simulink model "uz_FOC"  (R2021a)
settings: Solver=FixedStepDiscrete  StartTime=0.0  StopTime=50.0  FixedStep=0.00001  RelTol=1e-3  EnableMultiTasking=on
values from neighbouring files (symbols this model uses):
  d_d_TMS = 0.005    [uz_FOC_init.m]
  d_f_c = 100000    [uz_FOC_init.m]
  d_i_max = 10    [uz_FOC_init.m]
  d_i_min = -d_i_max    (= -10)    [uz_FOC_init.m]
  d_J_Coupling_M_E = 2e-6    (= 2e-06)    [uz_FOC_init.m]
  d_J_Coupling_M_Ms = 2e-20    [uz_FOC_init.m]
  d_J_Ms_L = d_J_Ms_M    (= 1.26363648e-05)    [uz_FOC_init.m]
  d_J_Ms_M = 0.5*0.5*((0.5*d_d_Ms)^4)*3.14*d_l_Ms*d_rho_Ms    (= 1.26363648e-05)    [uz_FOC_init.m]
  d_Ki_id = d_Kp_id/d_Tn_id    (= 2000)    [uz_FOC_init.m]
  d_Ki_iq = d_Kp_iq/d_Tn_iq    (= 2000)    [uz_FOC_init.m]
  d_Ki_n = d_Kp_n/d_Tn_n    (= 0.0864)    [uz_FOC_init.m]
  d_Kp_id = d_L_d / (4*1/d_f_c)    (= 6.75)    [uz_FOC_init.m]
  d_Kp_iq = d_L_q / (4*1/d_f_c)    (= 6.75)    [uz_FOC_init.m]
  d_Kp_n = 0.00864    [uz_FOC_init.m]
  d_L_d = d_L_ph_ph/2    (= 0.00027)    [uz_FOC_init.m]
  d_L_q = d_L_ph_ph/2    (= 0.00027)    [uz_FOC_init.m]
  d_p = 4    [uz_FOC_init.m]
  d_psi_pm = 0.0082    [uz_FOC_init.m]
  d_R_ph = d_R_ph_ph/2    (= 0.08)    [uz_FOC_init.m]
  d_y_max = 10    [uz_FOC_init.m]
  d_y_min = -d_y_max    (= -10)    [uz_FOC_init.m]
undefined symbols (not defined in the file or in its folder): i_d, i_q, para, u_d, u_q
libraries: fl_lib x44, nesl_utility x27, ee_lib x21, simulink x8, spsabctodq0Lib x2, spsdq0toabcLib x1, spsTriangleGeneratorLib x1
(part 2 of 3)

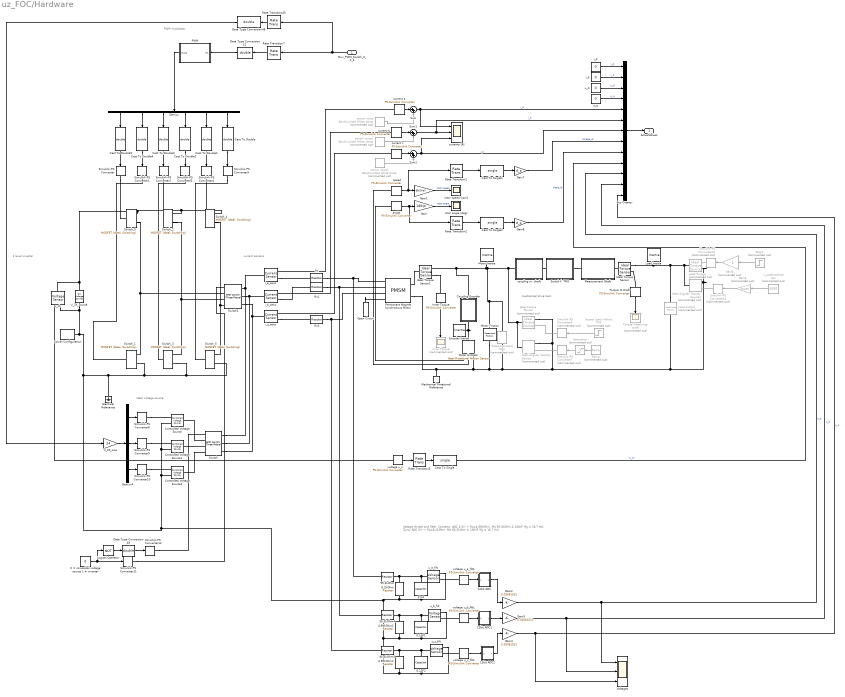
== system uz_FOC/Hardware ==
  note: PWM modulator
  note: 2 level inverter
  note: current sensors
  note: ideal voltage source
  note: Voltage divider and filter:
      | Concerto: ADC 3,3V -> RL=4,99kOhm. Mit 95,3kOhm & 100nF (fg = 16,7 Hz).
      | Zynq: ADC 5V -> RL=8,2kOhm. Mit 95,3kOhm & 100nF (fg = 16,7 Hz).
  note: mechanical drive train
  Mux_PWM_Switch_0_2_4 : Inport
  0 = sinusoidal voltage source 1 = inverter : Constant  Value=0
  0.1µF1 : ee_lib/Passive/Capacitor  cap_option=0  c=47 nF  Cvec=[ 1e-5 1e-6 ] F  Vvec=[ 0 10 ] V  CV_table_symmetry=1  f_vec=[1, 10] kHz  DFext_vec=[.8, 1.2]  C_tol=0.1  enable_C_tol=0  tol_distribution=1  nSigma=4  r=1e-18 Ohm  g=0 1/Ohm  averaging_period=0 s  enable_operating_limits=0  operating_limit_action=2  max_working_voltage_range=[ -25 25 ] V  power_rating=1 W  enable_faults=0  fault_action=1  Cscale_faulted=100  R_faulted=0.001 Ohm  G_faulted=0 1/Ohm  tau_fault=0.001 s  enable_temporal_fault=0  t_fault=1 s  enable_behavioral_fault=0  max_permissible_voltage_range=[ -100 100 ] V  t_fail_on_voltage=1 s  i_specify=off  i_priority=None  i=0 A  i_nominal_specify=off  i_nominal_unit=A  i_nominal_value=1  v_specify=off  v_priority=None  v=0 V  v_nominal_specify=off  v_nominal_unit=V  v_nominal_value=1  vc_specify=on  vc_priority=High  vc=0 V  vc_nominal_specify=off  vc_nominal_unit=V  vc_nominal_value=1
  0.1µF2 : ee_lib/Passive/Capacitor  cap_option=0  c=47 nF  Cvec=[ 1e-5 1e-6 ] F  Vvec=[ 0 10 ] V  CV_table_symmetry=1  f_vec=[1, 10] kHz  DFext_vec=[.8, 1.2]  C_tol=0.1  enable_C_tol=0  tol_distribution=1  nSigma=4  r=1e-18 Ohm  g=0 1/Ohm  averaging_period=0 s  enable_operating_limits=0  operating_limit_action=2  max_working_voltage_range=[ -25 25 ] V  power_rating=1 W  enable_faults=0  fault_action=1  Cscale_faulted=100  R_faulted=0.001 Ohm  G_faulted=0 1/Ohm  tau_fault=0.001 s  enable_temporal_fault=0  t_fault=1 s  enable_behavioral_fault=0  max_permissible_voltage_range=[ -100 100 ] V  t_fail_on_voltage=1 s  i_specify=off  i_priority=None  i=0 A  i_nominal_specify=off  i_nominal_unit=A  i_nominal_value=1  v_specify=off  v_priority=None  v=0 V  v_nominal_specify=off  v_nominal_unit=V  v_nominal_value=1  vc_specify=on  vc_priority=High  vc=0 V  vc_nominal_specify=off  vc_nominal_unit=V  vc_nominal_value=1
  12bit ADC : MATLAB Function  TreatAsAtomicUnit=on
  12bit ADC1 : MATLAB Function  TreatAsAtomicUnit=on
  12bit ADC2 : MATLAB Function  TreatAsAtomicUnit=on
  4,99kOhm1 : ee_lib/Passive/Resistor  R=8200 Ohm  R_tol=0.1  enable_R_tol=0  tol_distribution=1  nSigma=4  enable_operating_limits=0  operating_limit_action=2  max_working_voltage=100 V  power_rating=1 W  enable_faults=0  fault_action=1  R_faulted=Inf Ohm  enable_temporal_fault=0  t_fault=1 s  enable_behavioral_fault=0  max_permissible_current=1 A  t_fail_on_current=1 s  noise_mode=0  sample_time=0.001 s  repeatability=1  auto_seed=3032444857  user_seed=0  Tdevice=25 degC  alpha=3.93e-3 1/K  Tmeas=25 degC  thermal_mass=100 J/K  power_derating_T1=70 degC  power_derating_T2=155 degC  operating_temperature_range_vec=[-50, 150] degC  temperature_specify=off  temperature_priority=High  temperature=298.15 K  temperature_nominal_specify=off  temperature_nominal_unit=K  temperature_nominal_value=1
  4,99kOhm2 : ee_lib/Passive/Resistor  R=8200 Ohm  R_tol=0.1  enable_R_tol=0  tol_distribution=1  nSigma=4  enable_operating_limits=0  operating_limit_action=2  max_working_voltage=100 V  power_rating=1 W  enable_faults=0  fault_action=1  R_faulted=Inf Ohm  enable_temporal_fault=0  t_fault=1 s  enable_behavioral_fault=0  max_permissible_current=1 A  t_fail_on_current=1 s  noise_mode=0  sample_time=0.001 s  repeatability=1  auto_seed=136721035  user_seed=0  Tdevice=25 degC  alpha=3.93e-3 1/K  Tmeas=25 degC  thermal_mass=100 J/K  power_derating_T1=70 degC  power_derating_T2=155 degC  operating_temperature_range_vec=[-50, 150] degC  temperature_specify=off  temperature_priority=High  temperature=298.15 K  temperature_nominal_specify=off  temperature_nominal_unit=K  temperature_nominal_value=1
  47nF : ee_lib/Passive/Capacitor  cap_option=0  c=47 nF  Cvec=[ 1e-5 1e-6 ] F  Vvec=[ 0 10 ] V  CV_table_symmetry=1  f_vec=[1, 10] kHz  DFext_vec=[.8, 1.2]  C_tol=0.1  enable_C_tol=0  tol_distribution=1  nSigma=4  r=1e-20 Ohm  g=0 1/Ohm  averaging_period=0 s  enable_operating_limits=0  operating_limit_action=2  max_working_voltage_range=[ -25 25 ] V  power_rating=1 W  enable_faults=0  fault_action=1  Cscale_faulted=100  R_faulted=0.001 Ohm  G_faulted=0 1/Ohm  tau_fault=0.001 s  enable_temporal_fault=0  t_fault=1 s  enable_behavioral_fault=0  max_permissible_voltage_range=[ -100 100 ] V  t_fail_on_voltage=1 s  i_specify=off  i_priority=None  i=0 A  i_nominal_specify=off  i_nominal_unit=A  i_nominal_value=1  v_specify=off  v_priority=None  v=0 V  v_nominal_specify=off  v_nominal_unit=V  v_nominal_value=1  vc_specify=on  vc_priority=High  vc=0 V  vc_nominal_specify=off  vc_nominal_unit=V  vc_nominal_value=1
  8,2kOhm : ee_lib/Passive/Resistor  R=8200 Ohm  R_tol=0.1  enable_R_tol=0  tol_distribution=1  nSigma=4  enable_operating_limits=0  operating_limit_action=2  max_working_voltage=100 V  power_rating=1 W  enable_faults=0  fault_action=1  R_faulted=Inf Ohm  enable_temporal_fault=0  t_fault=1 s  enable_behavioral_fault=0  max_permissible_current=1 A  t_fail_on_current=1 s  noise_mode=0  sample_time=0.001 s  repeatability=1  auto_seed=1189375164  user_seed=0  Tdevice=25 degC  alpha=3.93e-3 1/K  Tmeas=25 degC  thermal_mass=100 J/K  power_derating_T1=70 degC  power_derating_T2=155 degC  operating_temperature_range_vec=[-50, 150] degC  temperature_specify=off  temperature_priority=High  temperature=298.15 K  temperature_nominal_specify=off  temperature_nominal_unit=K  temperature_nominal_value=1
  95,3kOhm : ee_lib/Passive/Resistor  R=95300 Ohm  R_tol=0.1  enable_R_tol=0  tol_distribution=1  nSigma=4  enable_operating_limits=0  operating_limit_action=2  max_working_voltage=100 V  power_rating=1 W  enable_faults=0  fault_action=1  R_faulted=Inf Ohm  enable_temporal_fault=0  t_fault=1 s  enable_behavioral_fault=0  max_permissible_current=1 A  t_fail_on_current=1 s  noise_mode=0  sample_time=0.001 s  repeatability=1  auto_seed=198304613  user_seed=0  Tdevice=25 degC  alpha=3.93e-3 1/K  Tmeas=25 degC  thermal_mass=100 J/K  power_derating_T1=70 degC  power_derating_T2=155 degC  operating_temperature_range_vec=[-50, 150] degC  temperature_specify=off  temperature_priority=High  temperature=298.15 K  temperature_nominal_specify=off  temperature_nominal_unit=K  temperature_nominal_value=1
  95,3kOhm4 : ee_lib/Passive/Resistor  R=95300 Ohm  R_tol=0.1  enable_R_tol=0  tol_distribution=1  nSigma=4  enable_operating_limits=0  operating_limit_action=2  max_working_voltage=100 V  power_rating=1 W  enable_faults=0  fault_action=1  R_faulted=Inf Ohm  enable_temporal_fault=0  t_fault=1 s  enable_behavioral_fault=0  max_permissible_current=1 A  t_fail_on_current=1 s  noise_mode=0  sample_time=0.001 s  repeatability=1  auto_seed=417177824  user_seed=0  Tdevice=25 degC  alpha=3.93e-3 1/K  Tmeas=25 degC  thermal_mass=100 J/K  power_derating_T1=70 degC  power_derating_T2=155 degC  operating_temperature_range_vec=[-50, 150] degC  temperature_specify=off  temperature_priority=High  temperature=298.15 K  temperature_nominal_specify=off  temperature_nominal_unit=K  temperature_nominal_value=1
  95,3kOhm5 : ee_lib/Passive/Resistor  R=95300 Ohm  R_tol=0.1  enable_R_tol=0  tol_distribution=1  nSigma=4  enable_operating_limits=0  operating_limit_action=2  max_working_voltage=100 V  power_rating=1 W  enable_faults=0  fault_action=1  R_faulted=Inf Ohm  enable_temporal_fault=0  t_fault=1 s  enable_behavioral_fault=0  max_permissible_current=1 A  t_fail_on_current=1 s  noise_mode=0  sample_time=0.001 s  repeatability=1  auto_seed=3536724442  user_seed=0  Tdevice=25 degC  alpha=3.93e-3 1/K  Tmeas=25 degC  thermal_mass=100 J/K  power_derating_T1=70 degC  power_derating_T2=155 degC  operating_temperature_range_vec=[-50, 150] degC  temperature_specify=off  temperature_priority=High  temperature=298.15 K  temperature_nominal_specify=off  temperature_nominal_unit=K  temperature_nominal_value=1
  Bus Creator : BusCreator  Inputs=13  OutDataTypeStr=Bus: ActualValues
  Cast To Double{,1..5} (6 alike) : DataTypeConversion  OutDataTypeStr=double
  Cast To Single : DataTypeConversion  OutDataTypeStr=single
  Cast To Single1 : DataTypeConversion  OutDataTypeStr=single
  Cast To Single2 : DataTypeConversion  OutDataTypeStr=single
  Controlled Voltage Source : fl_lib/Electrical/Electrical Sources/Controlled Voltage Source
  Controlled Voltage Source1 : fl_lib/Electrical/Electrical Sources/Controlled Voltage Source
  Controlled Voltage Source2 : fl_lib/Electrical/Electrical Sources/Controlled Voltage Source
  Coupling Encoder : Subsystem  Variant=on  VariantControlMode=label  LabelModeActiveChoice=TMS1
  Data Type Conversion12 : DataTypeConversion  OutDataTypeStr=double
  Data Type Conversion48 : DataTypeConversion  OutDataTypeStr=double
  Data Type Conversion49 : DataTypeConversion  OutDataTypeStr=double
  Demux : Demux  Outputs=6
  Demux4 : Demux  Outputs=3
  Electrical Reference : fl_lib/Electrical/Electrical Elements/Electrical Reference
  Encoder Inertia : fl_lib/Mechanical/Rotational Elements/Inertia  inertia=d_J_Encoder kg*m^2  num_ports=foundation.enum.numPorts2.one  w_specify=off  w_priority=High  w=0 rad/s  w_nominal_specify=off  w_nominal_unit=rad/s  w_nominal_value=1  t_specify=off  t_priority=None  t=0 N*m  t_nominal_specify=off  t_nominal_unit=N*m  t_nominal_value=1
  Gain : Gain  Gain=180/pi
  Gain1 : Gain  Gain=60/(2*pi)
  Gain2 : Gain  Gain=0.03081531  OutDataTypeStr=single
  Gain3 : Gain  Gain=0.03081531  OutDataTypeStr=single
  Gain4 : Gain  Gain=0.03081531  OutDataTypeStr=single
  Gain5 : Gain  Commented=on  Gain=-1
  Gain6 : Gain  Commented=on  Gain=2*pi/60
  Gain7 : Gain  Gain=d_p
  Gain8 : Gain  Gain=d_p
  Ideal Angular Velocity Source : fl_lib/Mechanical/Mechanical Sources/Ideal Angular Velocity Source  Commented=on
  Ideal Angular Velocity Source1 : fl_lib/Mechanical/Mechanical Sources/Ideal Angular Velocity Source  Commented=on
  Ideal Torque Sensor : fl_lib/Mechanical/Mechanical Sensors/Ideal Torque Sensor
  Ideal Torque Sensor1 : fl_lib/Mechanical/Mechanical Sensors/Ideal Torque Sensor
  Ideal Torque Source : fl_lib/Mechanical/Mechanical Sources/Ideal Torque Source  Commented=on
  Impact Load without TMS : Step  Commented=on  Time=0.05  SampleTime=0.0001
  Inner Torque : nesl_utility/PS-Simulink Converter  PhysicalDomain=network_engine_domain  SubClassName=ps_output  LeftPortType=input  RightPortType=output  PseudoPeriodic=off  Frequencies=[]  Unit=N*m  AffineConversion=off
      settings: SourceProductBaseCode=PW,SS
  "Inner Torque " : Scope  Commented=on
  Load Friction : fl_lib/Mechanical/Rotational Elements/Rotational Friction  Commented=on  brkwy_trq=d_M_stribeck N*m  brkwy_vel=d_v_stribeck rad/s  Col_trq=d_M_coulomb N*m  visc_coef=d_d_viscous N*m/(rad/s)  w_specify=on  w_priority=High  w=0 rad/s  w_nominal_specify=off  w_nominal_unit=rad/s  w_nominal_value=1  t_specify=on  t_priority=High  t=0 N*m  t_nominal_specify=off  t_nominal_unit=N*m  t_nominal_value=1
  Load Inertia : fl_lib/Mechanical/Rotational Elements/Inertia  inertia=d_J_Loadmachine kg*m^2  num_ports=foundation.enum.numPorts2.one  w_specify=off  w_priority=High  w=0 rad/s  w_nominal_specify=off  w_nominal_unit=rad/s  w_nominal_value=1  t_specify=off  t_priority=None  t=0 N*m  t_nominal_specify=off  t_nominal_unit=N*m  t_nominal_value=1
  Load Torque : fl_lib/Mechanical/Mechanical Sources/Ideal Torque Source  Commented=on
  Logical Operator : Logic  Operator=NOT  AllPortsSameDT=off  OutDataTypeStr=boolean
  Measurement Shaft : Subsystem  Variant=on  VariantControlMode=label  LabelModeActiveChoice=TMS1
  Mechanical Rotational Reference : fl_lib/Mechanical/Rotational Elements/Mechanical Rotational Reference
  Motor Encoder : fl_lib/Mechanical/Mechanical Sensors/Ideal Rotational Motion Sensor  wrap_angle=simscape.enum.onoff.off  offset=0 deg
  "Motor Inertia " : fl_lib/Mechanical/Rotational Elements/Inertia  inertia=d_J_m kg*m^2  num_ports=foundation.enum.numPorts2.one  w_specify=off  w_priority=High  w=0 rad/s  w_nominal_specify=off  w_nominal_unit=rad/s  w_nominal_value=1  t_specify=off  t_priority=None  t=0 N*m  t_nominal_specify=off  t_nominal_unit=N*m  t_nominal_value=1
  Motor Friction : fl_lib/Mechanical/Rotational Elements/Rotational Friction  brkwy_trq=d_M_stribeck N*m  brkwy_vel=d_v_stribeck rad/s  Col_trq=d_M_coulomb N*m  visc_coef=d_d_viscous N*m/(rad/s)  w_specify=on  w_priority=High  w=0 rad/s  w_nominal_specify=off  w_nominal_unit=rad/s  w_nominal_value=1  t_specify=on  t_priority=High  t=0 N*m  t_nominal_specify=off  t_nominal_unit=N*m  t_nominal_value=1
  Open Circuit : fl_lib/Electrical/Electrical Elements/Open Circuit  v_specify=off  v_priority=None  v=0 V  v_nominal_specify=off  v_nominal_unit=V  v_nominal_value=1
      settings: SourceProductBaseCode=SS
  PWM : Subsystem
  Permanent Magnet Synchronous Motor : ee_lib/Electromechanical/Permanent Magnet/PMSM  winding_type=ee.enum.statorconnection.wye  machine_param=ee.enum.pmsm.parameterization.constant  nPolePairs=d_p  pmflux_param=1  pm_flux_linkage=d_psi_pm Wb  torque_constant=0.18 N*m/A  back_emf_constant=0.18 V/(rad/s)  stator_param=1  Ld=d_L_d H  Lq=d_L_q H  idVec=[-200, 0, 200] A  iqVec=[-200, 0, 200] A  LdMatrix=0.0002 * ones(3, 3) H  LqMatrix=0.0002 * ones(3, 3) H  PmMatrix=0.1 * ones(3, 3) Wb  ktMatrix=0.18 * ones(3, 3) N*m/A  keMatrix=0.18 * ones(3, 3) V/(rad/s)  L0=d_L_0 H  Ls=0.0002 H  Lm=0.00002 H  Ms=0.00002 H  Rs=d_R_ph Ohm  zero_sequence=ee.enum.park.zerosequence.include  J=0 kg*m^2  lam=0 N*m/(rad/s)  axes_param=2  i_d_specify=off  i_d_priority=None  i_d=0 A  i_d_nominal_specify=off  i_d_nominal_unit=A  i_d_nominal_value=1  i_q_specify=off  i_q_priority=None  i_q=0 A  i_q_nominal_specify=off  i_q_nominal_unit=A  i_q_nominal_value=1  torque_specify=off  torque_priority=None  torque=0 N*m  torque_nominal_specify=off  torque_nominal_unit=N*m  torque_nominal_value=1  angular_velocity_specify=on  angular_velocity_priority=None  angular_velocity=0 rpm  angular_velocity_nominal_specify=off  angular_velocity_nominal_unit=rpm  angular_velocity_nominal_value=1  angular_position_specify=on  angular_position_priority=High  angular_position=0 deg  angular_position_nominal_specify=off  angular_position_nominal_unit=deg  angular_position_nominal_value=1  loss_param=ee.enum.ironloss.none  losses_oc=[0, 0, 0] W  losses_sc=[0, 0, 0] W  f_losses=60 Hz  Isc_losses=95 A  Tmeas=298.15 K  alpha=3.93e-3 1/K  alpha_flux=-0.001 1/K  stator_thermal_mass=100 J/K  rotor_thermal_mass=200 J/K  Rm_percent_rotor=90  Rd_percent_rotor=30  temperatureA_specify=off  temperatureA_priority=High  temperatureA=25 degC  temperatureA_nominal_specify=off  temperatureA_nominal_unit=degC  temperatureA_nominal_value=1  temperatureB_specify=off  temperatureB_priority=High  temperatureB=25 degC  temperatureB_nominal_specify=off  temperatureB_nominal_unit=degC  temperatureB_nominal_value=1  temperatureC_specify=off  temperatureC_priority=High  temperatureC=25 degC  temperatureC_nominal_specify=off  temperatureC_nominal_unit=degC  temperatureC_nominal_value=1  temperatureR_specify=off  temperatureR_priority=High  temperatureR=25 degC  temperatureR_nominal_specify=off  temperatureR_nominal_unit=degC  temperatureR_nominal_value=1
      settings: InternalSimscapePortConfiguration="{\"Bottom\":[],\"Left\":[{\"id\":\"a\",\"label\":\"a\",\"type\":\"foundation.electrical.electrical\"},{\"id\":\"b\",\"label\":\"b\",\"type\":\"foundation.electrical.electrical\"},{\"id\":\"c\",\"label\":\"c\",\"type\":\"foundation.electrical.electrical\"},{\"id\":\"n\",\"label\":\"n\",\"type\":\"foundation.electrical.electrical\"}],\"Right\":[{\"id\":\"R\",\"label\":\"R\",\"type\":\"foundation.mechanical.rotational.rotational\"},{\"id\":\"C\",\"label\":\"C\",\"type\":\"foundation.mechanical.rotational.rotational\"}],\"Top\":[]}"
  Ramp : simulink/Sources/Ramp  Commented=on  slope=10000  start=0  InitialOutput=0
  Rate Transition{1..3,7,45} (5 alike) : RateTransition  OutPortSampleTime=0.00001
  Rc : ee_lib/Passive/Resistor  R=0.005 Ohm  R_tol=5  enable_R_tol=0  tol_distribution=1  nSigma=4  enable_operating_limits=0  operating_limit_action=2  max_working_voltage=100 V  power_rating=1 W  enable_faults=0  fault_action=1  R_faulted=Inf Ohm  enable_temporal_fault=0  t_fault=1 s  enable_behavioral_fault=0  max_permissible_current=1 A  t_fail_on_current=1 s  noise_mode=0  sample_time=0.001 s  repeatability=1  auto_seed=2984266212  user_seed=0  Tdevice=25 degC  alpha=3.93e-3 1/K  Tmeas=25 degC  thermal_mass=100 J/K  power_derating_T1=70 degC  power_derating_T2=155 degC  operating_temperature_range_vec=[-50, 150] degC  temperature_specify=off  temperature_priority=High  temperature=298.15 K  temperature_nominal_specify=off  temperature_nominal_unit=K  temperature_nominal_value=1
  Rc1 : ee_lib/Passive/Resistor  R=0.005 Ohm  R_tol=5  enable_R_tol=0  tol_distribution=1  nSigma=4  enable_operating_limits=0  operating_limit_action=2  max_working_voltage=100 V  power_rating=1 W  enable_faults=0  fault_action=1  R_faulted=Inf Ohm  enable_temporal_fault=0  t_fault=1 s  enable_behavioral_fault=0  max_permissible_current=1 A  t_fail_on_current=1 s  noise_mode=0  sample_time=0.001 s  repeatability=1  auto_seed=1361931897  user_seed=0  Tdevice=25 degC  alpha=3.93e-3 1/K  Tmeas=25 degC  thermal_mass=100 J/K  power_derating_T1=70 degC  power_derating_T2=155 degC  operating_temperature_range_vec=[-50, 150] degC  temperature_specify=off  temperature_priority=High  temperature=298.15 K  temperature_nominal_specify=off  temperature_nominal_unit=K  temperature_nominal_value=1
  Rc2 : ee_lib/Passive/Resistor  R=0.005 Ohm  R_tol=5  enable_R_tol=0  tol_distribution=1  nSigma=4  enable_operating_limits=0  operating_limit_action=2  max_working_voltage=100 V  power_rating=1 W  enable_faults=0  fault_action=1  R_faulted=Inf Ohm  enable_temporal_fault=0  t_fault=1 s  enable_behavioral_fault=0  max_permissible_current=1 A  t_fail_on_current=1 s  noise_mode=0  sample_time=0.001 s  repeatability=1  auto_seed=4081172623  user_seed=0  Tdevice=25 degC  alpha=3.93e-3 1/K  Tmeas=25 degC  thermal_mass=100 J/K  power_derating_T1=70 degC  power_derating_T2=155 degC  operating_temperature_range_vec=[-50, 150] degC  temperature_specify=off  temperature_priority=High  temperature=298.15 K  temperature_nominal_specify=off  temperature_nominal_unit=K  temperature_nominal_value=1
  Rotational Hard Stop : fl_lib/Mechanical/Rotational Elements/Rotational Hard Stop  Commented=on  upper_bnd=999999 rad  lower_bnd=0 rad  stiff_up=1e6 N*m/rad  stiff_low=1e6 N*m/rad  D_up=0.01 N*m/(rad/s)  D_low=0.01 N*m/(rad/s)  model=3  transition=0.001 rad  w_specify=off  w_priority=None  w=0 rad/s  w_nominal_specify=off  w_nominal_unit=rad/s  w_nominal_value=1  t_specify=off  t_priority=None  t=0 N*m  t_nominal_specify=off  t_nominal_unit=N*m  t_nominal_value=1  phi_specify=off  phi_priority=High  phi=0 rad  phi_nominal_specify=off  phi_nominal_unit=rad  phi_nominal_value=1
      settings: SourceProductBaseCode=SS
  Saturation : Saturate  Commented=on  UpperLimit=104.7/2
  Simulink-PS Converter{,1..5,8..12} (11 alike) : nesl_utility/Simulink-PS Converter  PhysicalDomain=network_engine_domain  SubClassName=ps_input  LeftPortType=input  RightPortType=output  PseudoPeriodic=off  Frequencies=[]  NoiseDistribution=none  NoiseParameters=[]  Unit=1  AffineConversion=off  FilteringAndDerivatives=zero  SimscapeFilterOrder=1  InputFilterTimeConstant=0.001  UdotUserProvided=1
      settings: SourceProductBaseCode=PW,SS
  Simulink-PS Converter13 : nesl_utility/Simulink-PS Converter  Commented=on  PhysicalDomain=network_engine_domain  SubClassName=ps_input  LeftPortType=input  RightPortType=output  PseudoPeriodic=off  Frequencies=[]  NoiseDistribution=none  NoiseParameters=[]  Unit=1  AffineConversion=off  FilteringAndDerivatives=zero  SimscapeFilterOrder=1  InputFilterTimeConstant=0.001  UdotUserProvided=1
      settings: SourceProductBaseCode=PW,SS
  Simulink-PS Converter14 : nesl_utility/Simulink-PS Converter  Commented=on  PhysicalDomain=network_engine_domain  SubClassName=ps_input  LeftPortType=input  RightPortType=output  PseudoPeriodic=off  Frequencies=[]  NoiseDistribution=none  NoiseParameters=[]  Unit=1  AffineConversion=off  FilteringAndDerivatives=zero  SimscapeFilterOrder=1  InputFilterTimeConstant=0.001  UdotUserProvided=1
      settings: SourceProductBaseCode=PW,SS
  Simulink-PS Converter6 : nesl_utility/Simulink-PS Converter  Commented=on  PhysicalDomain=network_engine_domain  SubClassName=ps_input  LeftPortType=input  RightPortType=output  PseudoPeriodic=off  Frequencies=[]  NoiseDistribution=none  NoiseParameters=[]  Unit=N*m  AffineConversion=off  FilteringAndDerivatives=zero  SimscapeFilterOrder=1  InputFilterTimeConstant=0.001  UdotUserProvided=1
      settings: SourceProductBaseCode=PW,SS
  Simulink-PS Converter7 : nesl_utility/Simulink-PS Converter  Commented=on  PhysicalDomain=network_engine_domain  SubClassName=ps_input  LeftPortType=input  RightPortType=output  PseudoPeriodic=off  Frequencies=[]  NoiseDistribution=none  NoiseParameters=[]  Unit=rad/s  AffineConversion=off  FilteringAndDerivatives=zero  SimscapeFilterOrder=1  InputFilterTimeConstant=0.001  UdotUserProvided=1
      settings: SourceProductBaseCode=PW,SS
  Solver Configuration : nesl_utility/Solver Configuration  PhysicalDomain=network_engine_domain  SubClassName=solver  LeftPortType=input  RightPortType=generic  Tones=[]  Harmonics=[]  SimulateNoise=off  Profile=off  UseLocalSampling=off  EnableSwitchedLinearOptims=on  FrequencyDomain=off  UseCCode=off  RelTol=0.001  AbsTol=1e-06  MinStep=1e-09  ToWorkspace=off  RevertToSquareIcSolve=off  NumHomotopyIterations=100  PhasorMode=off  PhasorModeNumHarmonics=1  DoDC=off  ResidualTolerance=1e-09  UseLocalSolver=on  LocalSolverChoice=NE_BACKWARD_EULER_ADVANCER  LocalSolverSampleTime=0.00001  DoFixedCost=on  MaxNonlinIter=3  MaxModeIter=2  ComputeImpulses=off  ImpulseIterations=2  LinearAlgebra=Sparse  EquationFormulation=NE_TIME_EF  DelaysMemoryBudget=1024  AutomaticFiltering=on  FilteringTimeConstant=0.001  PartitionStorageMethod=AS_NEEDED  PartitionMemoryBudget=1024  PartitionMethod=FAST
      settings: SourceProductBaseCode=PW,SS
  Step1 : Step  Commented=on  Time=0  After=0.2  SampleTime=0
  Sum : Sum  Inputs=|++  OutDataTypeStr=single
  Sum1 : Sum  Inputs=|++  OutDataTypeStr=single
  Sum2 : Sum  Inputs=|++  OutDataTypeStr=single
  Switch : ee_lib/Switches & Breakers/SPST Switch (Three-Phase)  R_closed=0.001 Ohm  G_open=1e-6 1/Ohm  threshold=0.1 V  i_vT_specify=off  i_vT_priority=None  i_vT=0 A  i_vT_nominal_specify=off  i_vT_nominal_unit=A  i_vT_nominal_value=1  I_specify=off  I_priority=None  I=[ 0 0 0 ] A  I_nominal_specify=off  I_nominal_unit=A  I_nominal_value=1  V_specify=off  V_priority=None  V=[ 0 0 0 ] V  V_nominal_specify=off  V_nominal_unit=V  V_nominal_value=1  i_a_specify=off  i_a_priority=None  i_a=0 A  i_a_nominal_specify=off  i_a_nominal_unit=A  i_a_nominal_value=1  v_a_specify=off  v_a_priority=None  v_a=0 V  v_a_nominal_specify=off  v_a_nominal_unit=V  v_a_nominal_value=1  i_b_specify=off  i_b_priority=None  i_b=0 A  i_b_nominal_specify=off  i_b_nominal_unit=A  i_b_nominal_value=1  v_b_specify=off  v_b_priority=None  v_b=0 V  v_b_nominal_specify=off  v_b_nominal_unit=V  v_b_nominal_value=1  i_c_specify=off  i_c_priority=None  i_c=0 A  i_c_nominal_specify=off  i_c_nominal_unit=A  i_c_nominal_value=1  v_c_specify=off  v_c_priority=None  v_c=0 V  v_c_nominal_specify=off  v_c_nominal_unit=V  v_c_nominal_value=1
      settings: SourceProductBaseCode=PS  InternalSimscapePortConfiguration="{\"Bottom\":[],\"Left\":[{\"id\":\"vT\",\"label\":\"vT\",\"type\":\"input\"},{\"id\":\"a1\",\"label\":\"a1\",\"type\":\"foundation.electrical.electrical\"},{\"id\":\"b1\",\"label\":\"b1\",\"type\":\"foundation.electrical.electrical\"},{\"id\":\"c1\",\"label\":\"c1\",\"type\":\"foundation.electrical.electrical\"}],\"Right\":[{\"id\":\"a2\",\"label\":\"a2\",\"type\":\"foundation.electrical.electrical\"},{\"id\":\"b2\",\"label\":\"b2\",\"type\":\"foundation.electrical.electrical\"},{\"id\":\"c2\",\"label\":\"c2\",\"type\":\"foundation.electrical.electrical\"}],\"Top\":[]}"
  Switch f. TMS : Subsystem  Variant=on  VariantControlMode=label  LabelModeActiveChoice=d_KupplZus==1
  Switch1 : ee_lib/Switches & Breakers/SPST Switch (Three-Phase)  R_closed=0.001 Ohm  G_open=1e-6 1/Ohm  threshold=0.1 V  i_vT_specify=off  i_vT_priority=None  i_vT=0 A  i_vT_nominal_specify=off  i_vT_nominal_unit=A  i_vT_nominal_value=1  I_specify=off  I_priority=None  I=[ 0 0 0 ] A  I_nominal_specify=off  I_nominal_unit=A  I_nominal_value=1  V_specify=off  V_priority=None  V=[ 0 0 0 ] V  V_nominal_specify=off  V_nominal_unit=V  V_nominal_value=1  i_a_specify=off  i_a_priority=None  i_a=0 A  i_a_nominal_specify=off  i_a_nominal_unit=A  i_a_nominal_value=1  v_a_specify=off  v_a_priority=None  v_a=0 V  v_a_nominal_specify=off  v_a_nominal_unit=V  v_a_nominal_value=1  i_b_specify=off  i_b_priority=None  i_b=0 A  i_b_nominal_specify=off  i_b_nominal_unit=A  i_b_nominal_value=1  v_b_specify=off  v_b_priority=None  v_b=0 V  v_b_nominal_specify=off  v_b_nominal_unit=V  v_b_nominal_value=1  i_c_specify=off  i_c_priority=None  i_c=0 A  i_c_nominal_specify=off  i_c_nominal_unit=A  i_c_nominal_value=1  v_c_specify=off  v_c_priority=None  v_c=0 V  v_c_nominal_specify=off  v_c_nominal_unit=V  v_c_nominal_value=1
      settings: SourceProductBaseCode=PS  InternalSimscapePortConfiguration="{\"Bottom\":[],\"Left\":[{\"id\":\"vT\",\"label\":\"vT\",\"type\":\"input\"},{\"id\":\"a1\",\"label\":\"a1\",\"type\":\"foundation.electrical.electrical\"},{\"id\":\"b1\",\"label\":\"b1\",\"type\":\"foundation.electrical.electrical\"},{\"id\":\"c1\",\"label\":\"c1\",\"type\":\"foundation.electrical.electrical\"}],\"Right\":[{\"id\":\"a2\",\"label\":\"a2\",\"type\":\"foundation.electrical.electrical\"},{\"id\":\"b2\",\"label\":\"b2\",\"type\":\"foundation.electrical.electrical\"},{\"id\":\"c2\",\"label\":\"c2\",\"type\":\"foundation.electrical.electrical\"}],\"Top\":[]}"
  Switch_{0..5} (6 alike) : ee_lib/Semiconductors & Converters/MOSFET (Ideal, Switching)  Rds=0.0077 Ohm  Goff=1e-6 1/Ohm  Vth=0.2 V  diode_param=2  diode_Vf=0.8 V  diode_Ron=0.001 Ohm  diode_Goff=1e-5 1/Ohm  diode_C=5e-8 F  diode_iRM=-235 A  diode_iF=300 A  diode_idot=-50 A/us  diode_trr_param=1  diode_trr_factor=3  diode_trr=15 us  diode_Qrr=1.5e+3 s*uA  thermal_loss_option=ee.enum.converters.thermalLossOption.constantvalues  Von_data=[0, 1.1, 1.3, 1.45, 1.75, 2.25, 2.7; 0, 1, 1.15, 1.35, 1.7, 2.35, 3] V  Eon_data=[0, .29, 1.43, 2.86, 5.71, 13.14, 22.86; 0, .57, 2.63, 5.14, 10.29, 20.57, 30.29] * 1e-3 J  Eoff_data=[0, .21, 1.07, 2.14, 4.29, 9.86, 17.14; 0, .43, 1.97, 3.86, 7.71, 15.43, 22.71] * 1e-3 J  Tj=[298.15, 398.15] K  Iout_data=[0, 10, 50, 100, 200, 400, 600] A  Eon_scalar=22.86e-3 J  Eoff_scalar=17.14e-3 J  Voff=300 V  Iout_scalar=600 A  diodeModelType=ee.enum.converters.diodeModelType.pwl  diode_IfMat=[.07, .12, .19, 1.75, 4.24, 7.32, 11.2; .16, .3, .72, 2.14, 4.02, 6.35, 9.12] A  diode_TjVec=[25, 125] degC  diode_VfVec=[.5, .7, .9, 1.3, 1.7, 2.1, 2.5] V  thermal_network_parameterization=ee.enum.thermalNetworkTopology.external  Rth=[.03, .2] K/W  Rth_Foster=[.03, .2] K/W  thermal_mass_parameterization=ee.enum.thermalNetwork.timeconstant  thermal_mass=[3, 25] J/K  thermal_mass_Foster=[33, 50] J/K  thermal_time_constant=[.1, 5] s  thermal_time_constant_Foster=[1, 10] s  thermal_mass_initial_temperatures=[25, 25] degC  junction_thermal_mass=0.1 J/K  vT_specify=off  vT_priority=None  vT=0 V  vT_nominal_specify=off  vT_nominal_unit=V  vT_nominal_value=1  Qj_specify=off  Qj_priority=None  Qj=0 W  Qj_nominal_specify=off  Qj_nominal_unit=W  Qj_nominal_value=1  junction_temperature_specify=off  junction_temperature_priority=None  junction_temperature=25 degC  junction_temperature_nominal_specify=off  junction_temperature_nominal_unit=degC  junction_temperature_nominal_value=1
  Torque Measuring- shaft : Scope  Commented=on
  Torque M.shaft : nesl_utility/PS-Simulink Converter  PhysicalDomain=network_engine_domain  SubClassName=ps_output  LeftPortType=input  RightPortType=output  PseudoPeriodic=off  Frequencies=[]  Unit=N*m  AffineConversion=off
      settings: SourceProductBaseCode=PW,SS
  U_ZK_sine : Gain  Gain=24
  U_ZK_source : fl_lib/Electrical/Electrical Sources/DC Voltage Source  v0=24 V
  Voltages : Scope  NumInputPorts=3
  angle : nesl_utility/PS-Simulink Converter  PhysicalDomain=network_engine_domain  SubClassName=ps_output  LeftPortType=input  RightPortType=output  PseudoPeriodic=off  Frequencies=[]  Unit=rad  AffineConversion=off
      settings: SourceProductBaseCode=PW,SS
  coupling m. shaft : Subsystem  Variant=on  VariantControlMode=label  LabelModeActiveChoice=TMS1
  current a : nesl_utility/PS-Simulink Converter  PhysicalDomain=network_engine_domain  SubClassName=ps_output  LeftPortType=input  RightPortType=output  PseudoPeriodic=off  Frequencies=[]  Unit=A  AffineConversion=off
      settings: SourceProductBaseCode=PW,SS
  current b : nesl_utility/PS-Simulink Converter  PhysicalDomain=network_engine_domain  SubClassName=ps_output  LeftPortType=input  RightPortType=output  PseudoPeriodic=off  Frequencies=[]  Unit=A  AffineConversion=off
      settings: SourceProductBaseCode=PW,SS
  current c : nesl_utility/PS-Simulink Converter  PhysicalDomain=network_engine_domain  SubClassName=ps_output  LeftPortType=input  RightPortType=output  PseudoPeriodic=off  Frequencies=[]  Unit=A  AffineConversion=off
      settings: SourceProductBaseCode=PW,SS
  currents [A] : Scope  NumInputPorts=3
  i_a_sens : fl_lib/Electrical/Electrical Sensors/Current Sensor
  i_b_sens : fl_lib/Electrical/Electrical Sensors/Current Sensor
  i_c_sens : fl_lib/Electrical/Electrical Sensors/Current Sensor
  i_d : Constant  Value=0  OutDataTypeStr=single  SampleTime=1/d_f_c
  i_q : Constant  Value=0  OutDataTypeStr=single  SampleTime=1/d_f_c
  n_Loadmachine rpm : Constant  Commented=on  Value=4000
  rotor angle [deg] : Scope
  rotor speed [rpm] : Scope
  sensor noise : simulink/Sources/Band-Limited White Noise  Commented=on  Cov=[0.0000000001]  Ts=0.000001  seed=[23341]
  sensor noise1 : simulink/Sources/Band-Limited White Noise  Commented=on  Cov=[0.0000000001]  Ts=0.000001  seed=[43132]
  sensor noise2 : simulink/Sources/Band-Limited White Noise  Commented=on  Cov=[0.0000000001]  Ts=0.000001  seed=[12334]
  speed : nesl_utility/PS-Simulink Converter  PhysicalDomain=network_engine_domain  SubClassName=ps_output  LeftPortType=input  RightPortType=output  PseudoPeriodic=off  Frequencies=[]  Unit=rad/s  AffineConversion=off
      settings: SourceProductBaseCode=PW,SS
  u_a_filt : fl_lib/Electrical/Electrical Sensors/Voltage Sensor
      settings: LogSimulationData=on
  u_b_filt : fl_lib/Electrical/Electrical Sensors/Voltage Sensor
      settings: LogSimulationData=on
  u_c_filt : fl_lib/Electrical/Electrical Sensors/Voltage Sensor
      settings: LogSimulationData=on
  u_d : Constant  Value=0  OutDataTypeStr=single  SampleTime=1/d_f_c
  u_q : Constant  Value=0  OutDataTypeStr=single  SampleTime=1/d_f_c
  u_zk : fl_lib/Electrical/Electrical Sensors/Voltage Sensor
  voltage u_a_filt1 : nesl_utility/PS-Simulink Converter  PhysicalDomain=network_engine_domain  SubClassName=ps_output  LeftPortType=input  RightPortType=output  PseudoPeriodic=off  Frequencies=[]  Unit=V  AffineConversion=off
      settings: SourceProductBaseCode=PW,SS
  voltage u_b_filt1 : nesl_utility/PS-Simulink Converter  PhysicalDomain=network_engine_domain  SubClassName=ps_output  LeftPortType=input  RightPortType=output  PseudoPeriodic=off  Frequencies=[]  Unit=V  AffineConversion=off
      settings: SourceProductBaseCode=PW,SS
  voltage u_c_filt1 : nesl_utility/PS-Simulink Converter  PhysicalDomain=network_engine_domain  SubClassName=ps_output  LeftPortType=input  RightPortType=output  PseudoPeriodic=off  Frequencies=[]  Unit=V  AffineConversion=off
      settings: SourceProductBaseCode=PW,SS
  voltage u_s : nesl_utility/PS-Simulink Converter  PhysicalDomain=network_engine_domain  SubClassName=ps_output  LeftPortType=input  RightPortType=output  PseudoPeriodic=off  Frequencies=[]  Unit=V  AffineConversion=off
      settings: SourceProductBaseCode=PW,SS
  ActualValues : Outport  OutDataTypeStr=Bus: ActualValues
  wires:
  Mux_PWM_Switch_0_2_4/1 -> Rate Transition45/1, Rate Transition7/1
  sensor noise/1 -> Sum/2
  0 = sinusoidal voltage source 1 = inverter/1 -> Logical Operator/1, Simulink-PS Converter11/1
  voltage u_b_filt1/1 -> 12bit ADC1/1(u)
  Gain/1 -> rotor angle [deg]/1  "rotor angle"
  Demux4/2 -> Simulink-PS Converter9/1
  Sum/1 -> Bus Creator/5, currents [A]/1  "i_a"
  Gain1/1 -> rotor speed [rpm]/1  "rotor speed"
  Rate Transition45/1 -> Data Type Conversion48/1
  angle/1 -> Rate Transition2/1, Gain/1
  Data Type Conversion48/1 -> U_ZK_sine/1
  sensor noise2/1 -> Sum2/2
  12bit ADC/1(y) -> Gain2/1
  current a/1 -> Sum/1
  current b/1 -> Sum1/1
  Sum1/1 -> Bus Creator/6, currents [A]/2  "i_b"
  current c/1 -> Sum2/1
  PWM/1(Out1) -> Demux/1
  Data Type Conversion12/1 -> PWM/1(In1)
  Gain2/1 -> Bus Creator/11, Voltages/1  "u_a"
  Gain4/1 -> Bus Creator/13, Voltages/3  "u_c"
  voltage u_c_filt1/1 -> 12bit ADC2/1(u)
  voltage u_a_filt1/1 -> 12bit ADC/1(u)
  Inner Torque/1 -> "Inner Torque "/1
  speed/1 -> Rate Transition1/1, Gain1/1
  Torque M.shaft/1 -> Torque Measuring- shaft/1
  Saturation/1 -> Simulink-PS Converter7/1
  Step1/1 -> Gain5/1
  Gain3/1 -> Bus Creator/12, Voltages/2  "u_b"
  12bit ADC1/1(y) -> Gain3/1
  Impact Load without TMS/1 -> Simulink-PS Converter6/1
  Data Type Conversion49/1 -> Simulink-PS Converter12/1
  Logical Operator/1 -> Data Type Conversion49/1
  12bit ADC2/1(y) -> Gain4/1
  U_ZK_sine/1 -> Demux4/1
  Demux4/3 -> Simulink-PS Converter10/1
  sensor noise1/1 -> Sum1/2
  Demux4/1 -> Simulink-PS Converter8/1
  Sum2/1 -> Bus Creator/7, currents [A]/3  "i_c"
  Ramp/1 -> Saturation/1
  Rate Transition7/1 -> Data Type Conversion12/1
  Gain5/1 -> Simulink-PS Converter13/1
  Demux/6 -> Cast To Double/1
  Cast To Double/1 -> Simulink-PS Converter5/1
  Cast To Double5/1 -> Simulink-PS Converter/1
  Demux/1 -> Cast To Double5/1
  Demux/2 -> Cast To Double4/1
  Cast To Double4/1 -> Simulink-PS Converter1/1
  Demux/3 -> Cast To Double3/1
  Cast To Double3/1 -> Simulink-PS Converter2/1
  Demux/4 -> Cast To Double2/1
  Cast To Double2/1 -> Simulink-PS Converter3/1
  Demux/5 -> Cast To Double1/1
  Cast To Double1/1 -> Simulink-PS Converter4/1
  Cast To Single/1 -> Bus Creator/10  "U_zk"
  Rate Transition3/1 -> Cast To Single/1
  voltage u_s/1 -> Rate Transition3/1
  Rate Transition2/1 -> Cast To Single2/1
  Rate Transition1/1 -> Cast To Single1/1
  n_Loadmachine rpm/1 -> Gain6/1
  Gain6/1 -> Simulink-PS Converter14/1
  Cast To Single1/1 -> Gain7/1
  Gain7/1 -> Bus Creator/8  "omega_el"
  Gain8/1 -> Bus Creator/9  "theta_el"
  Cast To Single2/1 -> Gain8/1
  Bus Creator/1 -> ActualValues/1
  i_d/1 -> Bus Creator/1  "i_d"
  i_q/1 -> Bus Creator/2  "i_q"
  u_d/1 -> Bus Creator/3  "u_d"
  u_q/1 -> Bus Creator/4  "u_q"
  connections:
  Switch_0/RConn2 -- Switch1/LConn2 -- Switch_1/RConn1
  Switch/LConn2 -- Controlled Voltage Source/LConn1
  i_a_sens/RConn2 -- Rc/LConn1
  47nF/RConn1 -- Electrical Reference/LConn1 -- Switch_5/RConn2 -- Switch_3/RConn2 -- Switch_1/RConn2 -- u_zk/RConn2 -- U_ZK_source/RConn1 -- Solver Configuration/RConn1 -- Controlled Voltage Source/RConn2 -- Controlled Voltage Source1/RConn2 -- Controlled Voltage Source2/RConn2 -- 4,99kOhm2/RConn1 -- 0.1µF2/RConn1 -- u_c_filt/RConn2 -- u_b_filt/RConn2 -- 0.1µF1/RConn1 -- 4,99kOhm1/RConn1 -- 8,2kOhm/RConn1 -- u_a_filt/RConn2
  current c/LConn1 -- i_c_sens/RConn1
  Load Friction/RConn1 -- Ideal Angular Velocity Source1/RConn2 -- Load Torque/RConn2 -- Motor Encoder/RConn1 -- Permanent Magnet Synchronous Motor/RConn2 -- Mechanical Rotational Reference/LConn1 -- Motor Friction/RConn1 -- Rotational Hard Stop/RConn1 -- Ideal Torque Source/RConn2 -- Ideal Angular Velocity Source/RConn2
  Coupling Encoder/LConn1 -- Ideal Torque Source/LConn1 -- Ideal Angular Velocity Source/LConn1 -- coupling m. shaft/LConn1 -- Motor Friction/LConn1 -- Rotational Hard Stop/LConn1 -- "Motor Inertia "/LConn1 -- Ideal Torque Sensor1/RConn1
  u_c_filt/LConn1 -- 0.1µF2/LConn1 -- 4,99kOhm2/LConn1 -- 95,3kOhm5/RConn1
  95,3kOhm4/LConn1 -- Rc1/RConn1 -- Permanent Magnet Synchronous Motor/LConn2
  Switch/RConn2 -- Switch1/RConn2 -- i_b_sens/LConn1
  Switch/RConn3 -- Switch1/RConn3 -- i_c_sens/LConn1
  Simulink-PS Converter9/RConn1 -- Controlled Voltage Source1/RConn1
  Switch_4/RConn1 -- Switch_2/RConn1 -- u_zk/LConn1 -- U_ZK_source/LConn1 -- Switch_0/RConn1
  current b/LConn1 -- i_b_sens/RConn1
  Switch f. TMS/RConn1 -- Measurement Shaft/LConn1
  angle/LConn1 -- Motor Encoder/RConn3
  Measurement Shaft/RConn1 -- Ideal Torque Sensor/LConn1
  Load Friction/LConn1 -- Ideal Torque Sensor/RConn1 -- Load Inertia/LConn1 -- Ideal Angular Velocity Source1/LConn1 -- Load Torque/LConn1
  voltage u_s/LConn1 -- u_zk/RConn1
  Simulink-PS Converter1/RConn1 -- Switch_1/LConn1
  voltage u_a_filt1/LConn1 -- u_a_filt/RConn1
  Simulink-PS Converter4/RConn1 -- Switch_4/LConn1
  Simulink-PS Converter3/RConn1 -- Switch_3/LConn1
  Simulink-PS Converter10/RConn1 -- Controlled Voltage Source2/RConn1
  speed/LConn1 -- Motor Encoder/RConn2
  voltage u_c_filt1/LConn1 -- u_c_filt/RConn1
  current a/LConn1 -- i_a_sens/RConn1
  95,3kOhm/LConn1 -- Rc/RConn1 -- Permanent Magnet Synchronous Motor/LConn1
  Simulink-PS Converter8/RConn1 -- Controlled Voltage Source/RConn1
  Simulink-PS Converter14/RConn1 -- Ideal Angular Velocity Source1/RConn1
  Simulink-PS Converter5/RConn1 -- Switch_5/LConn1
  Switch_2/RConn2 -- Switch1/LConn3 -- Switch_3/RConn1
  Simulink-PS Converter2/RConn1 -- Switch_2/LConn1
  i_c_sens/RConn2 -- Rc2/LConn1
  95,3kOhm5/LConn1 -- Rc2/RConn1 -- Permanent Magnet Synchronous Motor/LConn3
  0.1µF1/LConn1 -- u_b_filt/LConn1 -- 4,99kOhm1/LConn1 -- 95,3kOhm4/RConn1
  Switch/RConn1 -- Switch1/RConn1 -- i_a_sens/LConn1
  Simulink-PS Converter12/RConn1 -- Switch/LConn1
  Simulink-PS Converter/RConn1 -- Switch_0/LConn1
  Switch/LConn4 -- Controlled Voltage Source2/LConn1
  Torque M.shaft/LConn1 -- Ideal Torque Sensor/RConn2
  Switch/LConn3 -- Controlled Voltage Source1/LConn1
  Ideal Torque Sensor1/LConn1 -- Permanent Magnet Synchronous Motor/RConn1
  Simulink-PS Converter6/RConn1 -- Ideal Torque Source/RConn1
  Open Circuit/LConn1 -- Permanent Magnet Synchronous Motor/LConn4
  u_a_filt/LConn1 -- 47nF/LConn1 -- 8,2kOhm/LConn1 -- 95,3kOhm/RConn1
  Coupling Encoder/RConn1 -- Encoder Inertia/LConn1 -- Motor Encoder/LConn1
  Simulink-PS Converter11/RConn1 -- Switch1/LConn1
  Switch_4/RConn2 -- Switch1/LConn4 -- Switch_5/RConn1
  Ideal Torque Sensor1/RConn2 -- Inner Torque/LConn1
  coupling m. shaft/RConn1 -- Switch f. TMS/LConn1
  Simulink-PS Converter7/RConn1 -- Ideal Angular Velocity Source/RConn1
  voltage u_b_filt1/LConn1 -- u_b_filt/RConn1
  Simulink-PS Converter13/RConn1 -- Load Torque/RConn1
  i_b_sens/RConn2 -- Rc1/LConn1

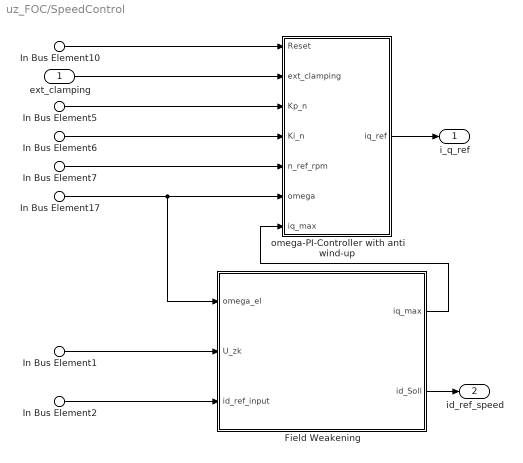
== system uz_FOC/SpeedControl ==
  ext_clamping : Inport
  In Bus Element5 : Inport  Port=2  PortName=conifg  Element=Kp_n
  In Bus Element6 : Inport  Port=2  PortName=conifg  Element=Ki_n
  In Bus Element7 : Inport  Port=2  PortName=conifg  Element=n_ref_rpm
  In Bus Element10 : Inport  Port=2  PortName=conifg  Element=IntegratorReset
  In Bus Element2 : Inport  Port=2  PortName=conifg  Element=id_ref
  In Bus Element17 : Inport  Port=3  PortName=ActualValues  Element=omega_el
  In Bus Element1 : Inport  Port=3  PortName=ActualValues  Element=U_zk
  Field Weakening : Subsystem
  omega-PI-Controller with anti wind-up : Subsystem
  i_q_ref : Outport  OutDataTypeStr=single
  id_ref_speed : Outport  Port=2  OutDataTypeStr=single
  wires:
  In Bus Element10/1 -> omega-PI-Controller with anti wind-up/1(Reset)
  In Bus Element7/1 -> omega-PI-Controller with anti wind-up/5(n_ref_rpm)
  In Bus Element6/1 -> omega-PI-Controller with anti wind-up/4(Ki_n)
  In Bus Element5/1 -> omega-PI-Controller with anti wind-up/3(Kp_n)
  ext_clamping/1 -> omega-PI-Controller with anti wind-up/2(ext_clamping)
  In Bus Element17/1 -> Field Weakening/1(omega_el), omega-PI-Controller with anti wind-up/6(omega)
  omega-PI-Controller with anti wind-up/1(iq_ref) -> i_q_ref/1
  In Bus Element1/1 -> Field Weakening/2(U_zk)
  Field Weakening/2(id_Soll) -> id_ref_speed/1
  Field Weakening/1(iq_max) -> omega-PI-Controller with anti wind-up/7(iq_max)
  In Bus Element2/1 -> Field Weakening/3(id_ref_input)

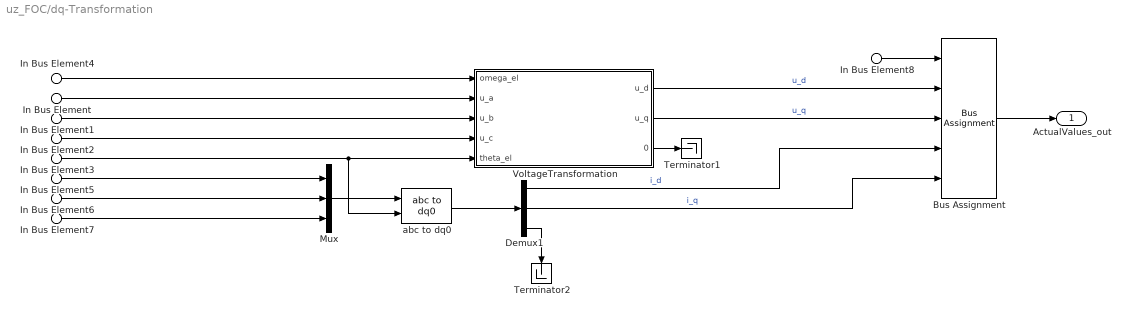
== system uz_FOC/dq-Transformation ==
  In Bus Element8 : Inport  PortName=ActualValues
  In Bus Element : Inport  PortName=ActualValues  Element=u_a
  In Bus Element1 : Inport  PortName=ActualValues  Element=u_b
  In Bus Element2 : Inport  PortName=ActualValues  Element=u_c
  In Bus Element3 : Inport  PortName=ActualValues  Element=theta_el
  In Bus Element4 : Inport  PortName=ActualValues  Element=omega_el
  In Bus Element5 : Inport  PortName=ActualValues  Element=i_a
  In Bus Element6 : Inport  PortName=ActualValues  Element=i_b
  In Bus Element7 : Inport  PortName=ActualValues  Element=i_c
  Bus Assignment : BusAssignment  AssignedSignals=u_d,u_q,i_d,i_q
  Demux1 : Demux  Outputs=3
  Mux : Mux  Inputs=3
  Terminator1 : Terminator
  Terminator2 : Terminator
  VoltageTransformation : Subsystem
  abc to dq0 : spsabctodq0Lib/abc to dq0  Alignment=Aligned with phase A axis
  ActualValues_out : Outport  OutDataTypeStr=Bus: ActualValues
  wires:
  In Bus Element5/1 -> Mux/1
  In Bus Element7/1 -> Mux/3
  In Bus Element4/1 -> VoltageTransformation/1(omega_el)
  In Bus Element1/1 -> VoltageTransformation/3(u_b)
  VoltageTransformation/3(0) -> Terminator1/1
  In Bus Element2/1 -> VoltageTransformation/4(u_c)
  Demux1/3 -> Terminator2/1
  In Bus Element3/1 -> abc to dq0/2, VoltageTransformation/5(theta_el)
  Mux/1 -> abc to dq0/1
  In Bus Element6/1 -> Mux/2
  In Bus Element/1 -> VoltageTransformation/2(u_a)
  abc to dq0/1 -> Demux1/1
  VoltageTransformation/1(u_d) -> Bus Assignment/2  "u_d"
  Bus Assignment/1 -> ActualValues_out/1
  In Bus Element8/1 -> Bus Assignment/1
  VoltageTransformation/2(u_q) -> Bus Assignment/3  "u_q"
  Demux1/1 -> Bus Assignment/4  "i_d"
  Demux1/2 -> Bus Assignment/5  "i_q"

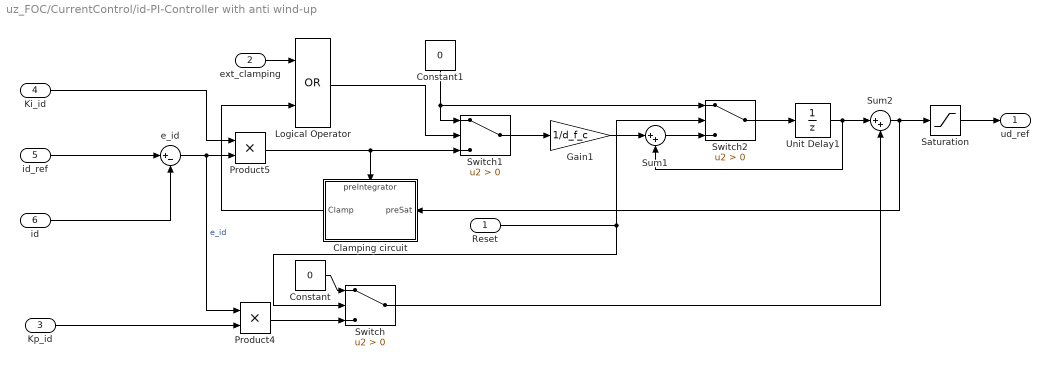
== system uz_FOC/CurrentControl/id-PI-Controller with anti wind-up ==
  Reset : Inport
  ext_clamping : Inport  Port=2
  Kp_id : Inport  Port=3
  Ki_id : Inport  Port=4
  id_ref : Inport  Port=5
  id : Inport  Port=6
  Clamping circuit : Subsystem
      settings: PortSchema="{\"entries\":[{\"content\":{\"sides\":[{\"content\":{\"connectorIds\":[\"In1\"]},\"type\":\"ConnectorPlacement.EquallySpacedRectSide\",\"uuid\":\"9b5eb3d3-336d-4b55-a615-0420b1cf4a48\"},{\"content\":{\"connectorIds\":[\"Out1\"],\"side\":\"RIGHT\"},\"type\":\"ConnectorPlacement.EquallySpacedRectSide\",\"uuid\":\"a73559ab-79dd-4c84-b45a-6a43ba4812e9\"},{\"content\":{\"connectorIds\":[\"In2\"],\"side\":\"TOP\"},\"type\":\"ConnectorPlacement.EquallySpacedRectSide\",\"uuid\":\"82c30f31-c271-4a2b-89be-8686aa9e20f3\"}]},\"type\":\"ConnectorPlacement.EquallySpacedConnector\",\"uuid\":\"376d2fe4-39b3-495b-8d80-8756076e2730\"}],\"packageUris\":[\"http://schema.mathworks.com/mf0/Connector/R2020b\"],\"version\":\"1.0\"}"
  Constant : Constant  Value=0  SampleTime=1/d_f_c
  Constant1 : Constant  Value=0  SampleTime=1/d_f_c
  Gain1 : Gain  Gain=1/d_f_c
  Logical Operator : Logic  Operator=OR  AllPortsSameDT=off  OutDataTypeStr=boolean
  Product4 : Product
  Product5 : Product
  Saturation : Saturate  UpperLimit=d_y_max  LowerLimit=d_y_min
  Sum1 : Sum  Inputs=|++  OutDataTypeStr=single
  Sum2 : Sum  Inputs=|++  OutDataTypeStr=single
  Switch : Switch  Criteria=u2 > Threshold
  Switch1 : Switch  Criteria=u2 > Threshold
  Switch2 : Switch  Criteria=u2 > Threshold
  Unit Delay1 : UnitDelay  SampleTime=-1  HasFrameUpgradeWarning=on
  e_id : Sum  Inputs=|+-
  ud_ref : Outport
  wires:
  Unit Delay1/1 -> Sum2/1, Sum1/2
  Kp_id/1 -> Product4/2
  id_ref/1 -> e_id/1
  Ki_id/1 -> Product5/1
  id/1 -> e_id/2
  e_id/1 -> Product5/2, Product4/1  "e_id"
  Switch/1 -> Sum2/2
  Logical Operator/1 -> Switch1/2
  ext_clamping/1 -> Logical Operator/1
  Sum2/1 -> Saturation/1, Clamping circuit/1(preSat)
  Clamping circuit/1(Clamp) -> Logical Operator/2
  Product5/1 -> Switch1/3, Clamping circuit/2(preIntegrator)
  Saturation/1 -> ud_ref/1
  Constant/1 -> Switch/1
  Product4/1 -> Switch/3
  Gain1/1 -> Sum1/1
  Constant1/1 -> Switch2/1, Switch1/1
  Reset/1 -> Switch/2, Switch2/2
  Sum1/1 -> Switch2/3
  Switch2/1 -> Unit Delay1/1
  Switch1/1 -> Gain1/1

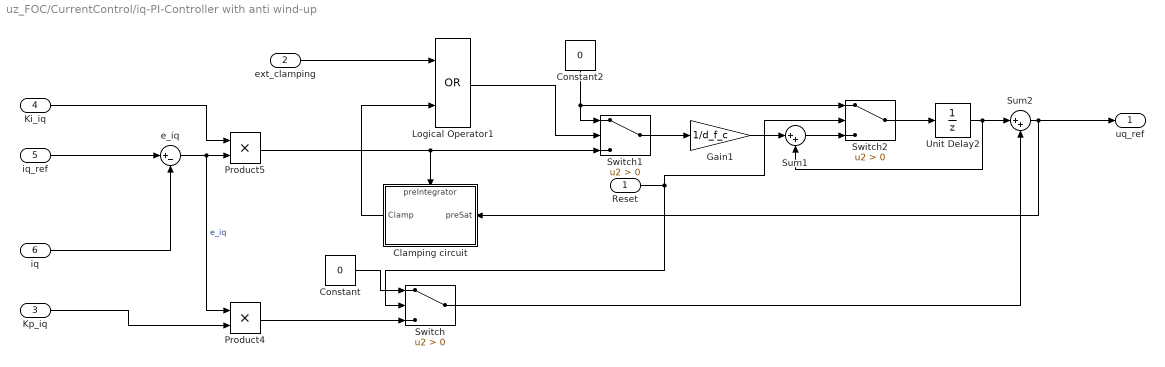
== system uz_FOC/CurrentControl/iq-PI-Controller with anti wind-up ==
  Reset : Inport
  ext_clamping : Inport  Port=2
  Kp_iq : Inport  Port=3
  Ki_iq : Inport  Port=4
  iq_ref : Inport  Port=5
  iq : Inport  Port=6
  Clamping circuit : Subsystem
      settings: PortSchema="{\"entries\":[{\"content\":{\"sides\":[{\"content\":{\"connectorIds\":[\"In1\"]},\"type\":\"ConnectorPlacement.EquallySpacedRectSide\",\"uuid\":\"9b5eb3d3-336d-4b55-a615-0420b1cf4a48\"},{\"content\":{\"connectorIds\":[\"Out1\"],\"side\":\"RIGHT\"},\"type\":\"ConnectorPlacement.EquallySpacedRectSide\",\"uuid\":\"a73559ab-79dd-4c84-b45a-6a43ba4812e9\"},{\"content\":{\"connectorIds\":[\"In2\"],\"side\":\"TOP\"},\"type\":\"ConnectorPlacement.EquallySpacedRectSide\",\"uuid\":\"82c30f31-c271-4a2b-89be-8686aa9e20f3\"}]},\"type\":\"ConnectorPlacement.EquallySpacedConnector\",\"uuid\":\"376d2fe4-39b3-495b-8d80-8756076e2730\"}],\"packageUris\":[\"http://schema.mathworks.com/mf0/Connector/R2020b\"],\"version\":\"1.0\"}"
  Constant : Constant  Value=0  SampleTime=1/d_f_c
  Constant2 : Constant  Value=0  SampleTime=1/d_f_c
  Gain1 : Gain  Gain=1/d_f_c
  Logical Operator1 : Logic  Operator=OR  AllPortsSameDT=off  OutDataTypeStr=boolean
  Product4 : Product
  Product5 : Product
  Sum1 : Sum  Inputs=|++  OutDataTypeStr=single
  Sum2 : Sum  Inputs=|++  OutDataTypeStr=single
  Switch : Switch  Criteria=u2 > Threshold
  Switch1 : Switch  Criteria=u2 > Threshold
  Switch2 : Switch  Criteria=u2 > Threshold
  Unit Delay2 : UnitDelay  SampleTime=-1  HasFrameUpgradeWarning=on
  e_iq : Sum  Inputs=|+-
  uq_ref : Outport
  wires:
  ext_clamping/1 -> Logical Operator1/1
  Kp_iq/1 -> Product4/2
  Ki_iq/1 -> Product5/1
  iq_ref/1 -> e_iq/1
  iq/1 -> e_iq/2
  e_iq/1 -> Product5/2, Product4/1  "e_iq"
  Unit Delay2/1 -> Sum2/1, Sum1/2
  Clamping circuit/1(Clamp) -> Logical Operator1/2
  Sum2/1 -> uq_ref/1, Clamping circuit/1(preSat)
  Switch/1 -> Sum2/2
  Constant/1 -> Switch/1
  Product4/1 -> Switch/3
  Switch2/1 -> Unit Delay2/1
  Gain1/1 -> Sum1/1
  Constant2/1 -> Switch2/1, Switch1/1
  Sum1/1 -> Switch2/3
  Product5/1 -> Switch1/3, Clamping circuit/2(preIntegrator)
  Switch1/1 -> Gain1/1
  Reset/1 -> Switch2/2, Switch/2
  Logical Operator1/1 -> Switch1/2

== system uz_FOC/CurrentControl/linear decouppling ==
  i_q : Inport
  i_d : Inport  Port=2
  omega_el : Inport  Port=3
  Gain : Gain  Gain=-d_L_q
  Gain4 : Gain  Gain=d_L_d
  Product : Product  SaturateOnIntegerOverflow=on
  Product1 : Product  SaturateOnIntegerOverflow=on
  Sum : Sum  Inputs=|++
  d_psi_pm : Constant  Value=d_psi_pm  OutDataTypeStr=Inherit: Inherit via back propagation  SampleTime=1/d_f_c
  u_d_vor : Outport  VectorParamsAs1DForOutWhenUnconnected=off
  u_q_vor : Outport  Port=2  VectorParamsAs1DForOutWhenUnconnected=off
  wires:
  i_q/1 -> Product/1
  Product1/1 -> u_q_vor/1
  Gain/1 -> Product/2
  Sum/1 -> Product1/1
  Product/1 -> u_d_vor/1
  omega_el/1 -> Gain/1, Product1/2
  Gain4/1 -> Sum/1
  d_psi_pm/1 -> Sum/2
  i_d/1 -> Gain4/1
